simulink model "Engine_Library"  (Simulink 7.7)
settings: Solver=ode45  StartTime=0.0  StopTime=10.0  RelTol=1e-3
PostLoadFcn:
  | %%% BEGIN C7_225HP_D_HF CODE %%%
  | % Import the data from Excel for a lookup table
  | data = xlsread('Engine_Specification.xlsx', 'C7_225HP_D');
  | % Row indices for lookup table
  | breakpoints1 = data(2:end,1)';
  | % Column indices for lookup table
  | breakpoints2 = data(1,2:end);
  | % Output values for lookup table
  | table_data = data(2:end,2:end);
  | Engine_C7_225HP_D_RPM_raw = table_data(:,1);
  | Engine_C7_225HP_D_Torque_raw = table_data(:,3);
  | Engine_C7_225HP_D_Power_raw = table_data(:,2);
  | Engine_C7_225HP_D_sfc_raw = table_data(:,4);
  | Engine_C7_225HP_D_ne_raw = table_data(:,5);
  | %%% END C7_225HP_D_HF CODE %%%%%% BEGIN C9_350HP_D_HF CODE %%%
  | % Import the data from Excel for a lookup table
  | data = xlsread('Engine_Specification.xlsx', 'C9_350HP_D');
  | % Row indices for lookup table
  | breakpoints1 = data(2:end,1)';
  | % Column indices for lookup table
  | breakpoints2 = data(1,2:end);
  | % Output values for lookup table
  | table_data = data(2:end,2:end);
  | Engine_C9_350HP_D_RPM_raw = table_data(:,1);
  | Engine_C9_350HP_D_Torque_raw = table_data(:,3);
  | Engine_C9_350HP_D_Power_raw = table_data(:,2);
  | Engine_C9_350HP_D_sfc_raw = table_data(:,4);
  | Engine_C9_350HP_D_ne_raw = table_data(:,5);
  | %%% END C9_350HP_D_HF CODE %%%%%% BEGIN C13_475HP_D_HF CODE %%%
  | % Import the data from Excel for a lookup table
  | data = xlsread('Engine_Specification.xlsx', 'C13_475HP_D');
  | % Row indices for lookup table
  | breakpoints1 = data(2:end,1)';
  | % Column indices for lookup table
  | breakpoints2 = data(1,2:end);
  | % Output values for lookup table
  | table_data = data(2:end,2:end);
  | Engine_C13_475HP_D_RPM_raw = table_data(:,1);
  | Engine_C13_475HP_D_Torque_raw = table_data(:,3);
  | Engine_C13_475HP_D_Power_raw = table_data(:,2);
  | Engine_C13_475HP_D_sfc_raw = table_data(:,4);
  | Engine_C13_475HP_D_ne_raw = table_data(:,5);
  | %%% END C13_475HP_D_HF CODE %%%%%% BEGIN C15_600HP_D_HF CODE %%%
  | % Import the data from Excel for a lookup table
  | data = xlsread('Engine_Specification.xlsx', 'C15_600HP_D');
  | % Row indices for lookup table
  | breakpoints1 = data(2:end,1)';
  | % Column indices for lookup table
  | breakpoints2 = data(1,2:end);
  | % Output values for lookup table
  | table_data = data(2:end,2:end);
  | Engine_C15_600HP_D_RPM_raw = table_data(:,1);
  | Engine_C15_600HP_D_Torque_raw = table_data(:,3);
  | Engine_C15_600HP_D_Power_raw = table_data(:,2);
  | Engine_C15_600HP_D_sfc_raw = table_data(:,4);
  | Engine_C15_600HP_D_ne_raw = table_data(:,5);
  | %%% END C15_600HP_D_HF CODE %%%%%% BEGIN C7_230HP_LEFT CODE %%%
  | % Import the data from Excel for a lookup table
  | data = xlsread('Engine_Specification.xlsx', 'C7_230HP_LEFT');
  | % Row indices for lookup table
  | breakpoints1 = data(2:end,1)';
  | % Column indices for lookup table
  | breakpoints2 = data(1,2:end);
  | % Output values for lookup table
  | table_data = data(2:end,2:end);
  | Engine_C7_230HP_LEFT_RPM_raw = table_data(:,1);
  | Engine_C7_230HP_LEFT_Torque_raw = table_data(:,3);
  | Engine_C7_230HP_LEFT_Power_raw = table_data(:,2);
  | Engine_C7_230HP_LEFT_sfc_raw = table_data(:,4);
  | Engine_C7_230HP_LEFT_ne_raw = table_data(:,5);
  | %%% END C7_230HP_LEFT CODE %%%%%% BEGIN C9_COM_350HP CODE %%%
  | % Import the data from Excel for a lookup table
  | data = xlsread('Engine_Specification.xlsx', 'C9_COM_350HP');
  | % Row indices for lookup table
  | breakpoints1 = data(2:end,1)';
  | % Column indices for lookup table
  | breakpoints2 = data(1,2:end);
  | % Output values for lookup table
  | table_data = data(2:end,2:end);
  | Engine_C9_COM_350HP_RPM_raw = table_data(:,1);
  | Engine_C9_COM_350HP_Torque_raw = table_data(:,3);
  | Engine_C9_COM_350HP_Power_raw = table_data(:,2);
  | Engine_C9_COM_350HP_sfc_raw = table_data(:,4);
  | %%% END C9_COM_350HP CODE %%%%%% BEGIN C13_COM_430HP CODE %%%
  | % Import the data from Excel for a lookup table
  | data = xlsread('Engine_Specification.xlsx', 'C13_COM_430HP');
  | % Row indices for lookup table
  | breakpoints1 = data(2:end,1)';
  | % Column indices for lookup table
  | breakpoints2 = data(1,2:end);
  | % Output values for lookup table
  | table_data = data(2:end,2:end);
  | Engine_C13_COM_430HP_RPM_raw = table_data(:,1);
  | Engine_C13_COM_430HP_Torque_raw = table_data(:,3);
  | Engine_C13_COM_430HP_Power_raw = table_data(:,2);
  | Engine_C13_COM_430HP_sfc_raw = table_data(:,4);
  | %%% END C13_COM_430HP CODE %%%
libraries: simulink x3
settings Model: Creator=Zsolt  LastModifiedBy=jscott
settings HardwareCC: TargetIntDivRoundTo=Zero  TargetEndianess=LittleEndian  TargetHWDeviceType=MATLAB Host  ProdEqTarget=off
settings RTWCC: SystemTargetFile=rsim.tlc  TemplateMakefile=rsim_default_tmf  Description=Rapid Simulation Target  ProcessScript=rsim_make_rtw_hook
settings RSimTargetCC: TargetFunctionLibrary=ANSI_C  ERTMultiwordTypeDef=System defined  FunctionExecutionProfile=off  CodeExecutionProfiling=off  ERTCodeCoverageTool=None  ERTMultiwordLength=256  IsPILTarget=off  EnableShiftOperators=on  PortableWordSizes=off

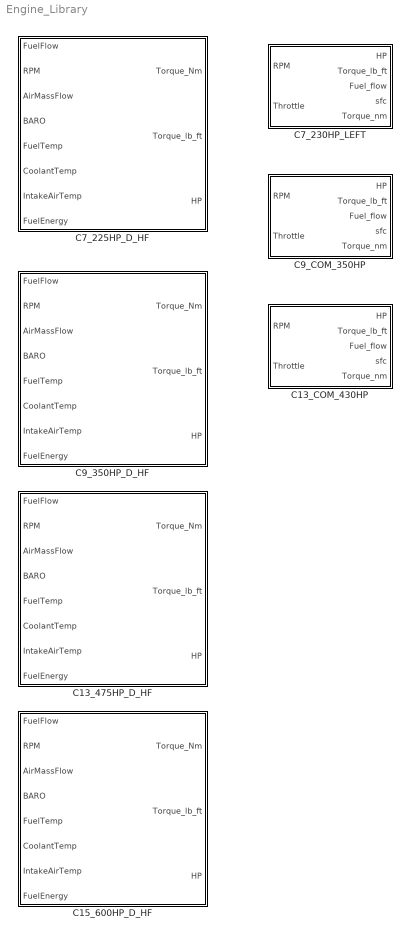
== system Engine_Library ==
  C13_475HP_D_HF : Subsystem
  C13_COM_430HP : Subsystem
  C15_600HP_D_HF : Subsystem
  C7_225HP_D_HF : Subsystem
  C7_230HP_LEFT : Subsystem
  C9_350HP_D_HF : Subsystem
  C9_COM_350HP : Subsystem

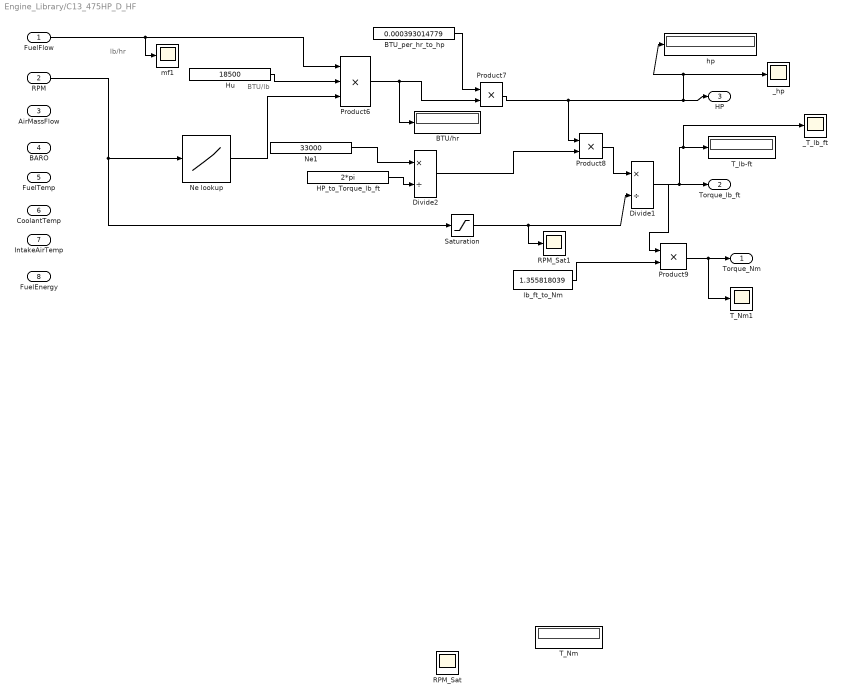
== system Engine_Library/C13_475HP_D_HF ==
  note: lb/hr
  note: BTU/lb
  FuelFlow : Inport
  RPM : Inport  Port=2
  AirMassFlow : Inport  Port=3
  BARO : Inport  Port=4
  FuelTemp : Inport  Port=5
  CoolantTemp : Inport  Port=6
  IntakeAirTemp : Inport  Port=7
  FuelEnergy : Inport  Port=8
  BTU/hr : Display
  BTU_per_hr_to_hp : Constant  Value=0.000393014779
  Divide1 : Product  Inputs=*/
  Divide2 : Product  Inputs=*/
  HP_to_Torque_lb_ft : Constant  Value=2*pi
  Hu : Constant  Value=18500
  Ne lookup : Lookup  InputValues=Engine_C13_475HP_D_RPM_raw  Table=Engine_C13_475HP_D_ne_raw
  Ne1 : Constant  Value=33000
  Product6 : Product  Inputs=3  RndMeth=Zero
  Product7 : Product  RndMeth=Zero
  Product8 : Product  RndMeth=Zero
  Product9 : Product  RndMeth=Zero
  RPM_Sat : Scope
      settings: TimeRange=100  SaveName=ScopeData4
  RPM_Sat1 : Scope
      settings: TimeRange=100  SaveName=ScopeData7
  Saturation : Saturate  UpperLimit=2100  LowerLimit=600
  T_Nm : Display
  T_Nm1 : Scope
      settings: TimeRange=100  SaveName=ScopeData6
  T_lb-ft : Display
  _T_lb_ft : Scope
      settings: SaveName=ScopeData5
  _hp : Scope
      settings: SaveName=ScopeData3
  hp : Display
  lb_ft_to_Nm : Constant  Value=1.355818039
  mf1 : Scope
      settings: SaveName=ScopeData8
  Torque_Nm : Outport
  Torque_lb_ft : Outport  Port=2
  HP : Outport  Port=3
  wires:
  FuelFlow/1 -> Product6/1, mf1/1
  Hu/1 -> Product6/2
  HP_to_Torque_lb_ft/1 -> Divide2/2
  Ne1/1 -> Divide2/1
  BTU_per_hr_to_hp/1 -> Product7/1
  Product7/1 -> Product8/1, HP/1, _hp/1, hp/1
  Product6/1 -> Product7/2, BTU/hr/1
  Divide2/1 -> Product8/2
  lb_ft_to_Nm/1 -> Product9/2
  Divide1/1 -> Torque_lb_ft/1, Product9/1, T_lb-ft/1, _T_lb_ft/1
  Product8/1 -> Divide1/1
  Saturation/1 -> Divide1/2, RPM_Sat1/1
  Product9/1 -> Torque_Nm/1, T_Nm1/1
  RPM/1 -> Saturation/1, Ne lookup/1
  Ne lookup/1 -> Product6/3

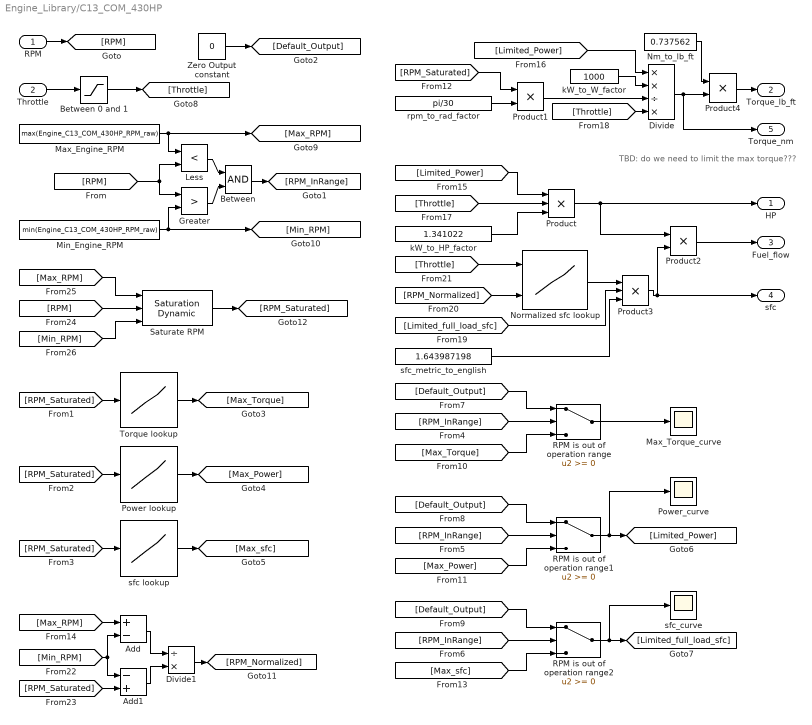
== system Engine_Library/C13_COM_430HP ==
  note: TBD: do we need to limit the max torque???
  RPM : Inport
  Throttle : Inport  Port=2
  Add : Sum  Inputs=+-
  Add1 : Sum  Inputs=-+
  Between : Logic  AllPortsSameDT=off  OutDataTypeStr=boolean
  Between 0 and 1 : Saturate  UpperLimit=1  LowerLimit=0
  Divide : Product  Inputs=**/*
  Divide1 : Product  Inputs=/*
  Greater : RelationalOperator  Operator=>  OutDataTypeStr=boolean
  Less : RelationalOperator  Operator=<  OutDataTypeStr=boolean
  Max_Engine_RPM : Constant  Value=max(Engine_C13_COM_430HP_RPM_raw)
  Max_Torque_curve : Scope
      settings: TimeRange=10  YMin=500  YMax=1000
  Min_Engine_RPM : Constant  Value=min(Engine_C13_COM_430HP_RPM_raw)
  Nm_to_lb_ft : Constant  Value=0.737562
  Normalized sfc lookup : Lookup2D  RowIndex=[0,0.25,0.5,0.75,1]  ColumnIndex=[0,0.25,0.5,0.75,1]  Table=[ 1.3562, 1.1898, 1.0652, 1.0227, 1.0000; 1.3918, 1.2098, 1.0718, 1.0316, 1.0000; 1.4074, 1.2248, 1.0865, 1.0461, 1.0000; 1.4502, 1.2557, 1.1108, 1.0540, 1.0000; 1.4127, 1.2404, 1.1120, 1.0628, 1.0000]'  LookUpMeth=Interpolation-Use End Values
  Power lookup : Lookup  InputValues=Engine_C13_COM_430HP_RPM_raw  Table=Engine_C13_COM_430HP_Power_raw
  Power_curve : Scope
      settings: TimeRange=10  YMin=50  YMax=250
  Product : Product  Inputs=3  RndMeth=Zero
  Product1 : Product  RndMeth=Zero
  Product2 : Product  RndMeth=Zero
  Product3 : Product  Inputs=3  RndMeth=Zero
  Product4 : Product  RndMeth=Zero
  RPM is out of operation range : Switch
  RPM is out of operation range1 : Switch
  RPM is out of operation range2 : Switch
  Saturate RPM : simulink/Discontinuities/Saturation Dynamic  SystemSampleTime=-1  OutMin=[]  OutMax=[]  OutDataTypeStr=Inherit: Same as second input  OutDataType=fixdt(1, 16)  OutScaling=2^-10  DoSatur=off
  Torque lookup : Lookup  InputValues=Engine_C13_COM_430HP_RPM_raw  Table=Engine_C13_COM_430HP_Torque_raw
  Zero Output constant : Constant  Value=0
  kW_to_HP_factor : Constant  Value=1.341022
  kW_to_W_factor : Constant  Value=1000
  rpm_to_rad_factor : Constant  Value=pi/30
  sfc lookup : Lookup  InputValues=Engine_C13_COM_430HP_RPM_raw  Table=Engine_C13_COM_430HP_sfc_raw
  sfc_curve : Scope
      settings: TimeRange=10  YMin=40  YMax=120  SaveName=ScopeData2
  sfc_metric_to_english : Constant  Value=1.643987198
  HP : Outport
  Torque_lb_ft : Outport  Port=2
  Fuel_flow : Outport  Port=3
  sfc : Outport  Port=4
  Torque_nm : Outport  Port=5
  wires:
  Power lookup/1 -> [Max_Power]
  sfc lookup/1 -> [Max_sfc]
  Torque lookup/1 -> [Max_Torque]
  Max_Engine_RPM/1 -> Less/1, [Max_RPM]
  RPM is out of operation range/1 -> Max_Torque_curve/1
  Throttle/1 -> Between 0 and 1/1
  kW_to_HP_factor/1 -> Product/3
  Product/1 -> HP/1, Product2/1
  rpm_to_rad_factor/1 -> Product1/2
  Product1/1 -> Divide/3
  kW_to_W_factor/1 -> Divide/2
  Product2/1 -> Fuel_flow/1
  RPM/1 -> [RPM]
  [RPM] -> Less/2, Greater/1
  [RPM_Saturated] -> Torque lookup/1
  [RPM_Saturated] -> Power lookup/1
  [RPM_Saturated] -> sfc lookup/1
  [RPM_InRange] -> RPM is out of operation range/2
  [RPM_InRange] -> RPM is out of operation range1/2
  [RPM_InRange] -> RPM is out of operation range2/2
  Zero Output constant/1 -> [Default_Output]
  [Default_Output] -> RPM is out of operation range/1
  [Default_Output] -> RPM is out of operation range1/1
  [Default_Output] -> RPM is out of operation range2/1
  [Max_Torque] -> RPM is out of operation range/3
  [Max_Power] -> RPM is out of operation range1/3
  [RPM_Saturated] -> Product1/1
  [Max_sfc] -> RPM is out of operation range2/3
  RPM is out of operation range1/1 -> [Limited_Power], Power_curve/1
  RPM is out of operation range2/1 -> [Limited_full_load_sfc], sfc_curve/1
  [Limited_Power] -> Product/1
  [Limited_Power] -> Divide/1
  Between 0 and 1/1 -> [Throttle]
  [Throttle] -> Product/2
  [Throttle] -> Divide/4
  Min_Engine_RPM/1 -> Greater/2, [Min_RPM]
  Less/1 -> Between/1
  Greater/1 -> Between/2
  Between/1 -> [RPM_InRange]
  Normalized sfc lookup/1 -> Product3/1
  [Limited_full_load_sfc] -> Product3/2
  sfc_metric_to_english/1 -> Product3/3
  Product3/1 -> sfc/1, Product2/2
  [Max_RPM] -> Add/1
  [Min_RPM] -> Add/2, Add1/1
  [RPM_Saturated] -> Add1/2
  Add/1 -> Divide1/1
  Add1/1 -> Divide1/2
  Divide1/1 -> [RPM_Normalized]
  [Throttle] -> Normalized sfc lookup/1
  [RPM_Normalized] -> Normalized sfc lookup/2
  [RPM] -> Saturate RPM/2
  [Max_RPM] -> Saturate RPM/1
  [Min_RPM] -> Saturate RPM/3
  Saturate RPM/1 -> [RPM_Saturated]
  Divide/1 -> Torque_nm/1, Product4/2
  Product4/1 -> Torque_lb_ft/1
  Nm_to_lb_ft/1 -> Product4/1

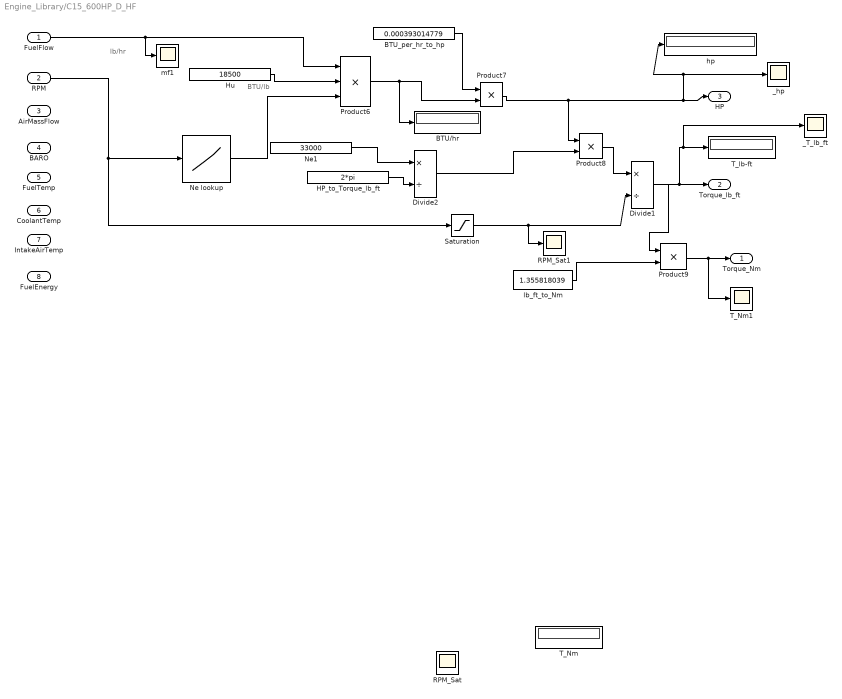
== system Engine_Library/C15_600HP_D_HF ==
  note: lb/hr
  note: BTU/lb
  FuelFlow : Inport
  RPM : Inport  Port=2
  AirMassFlow : Inport  Port=3
  BARO : Inport  Port=4
  FuelTemp : Inport  Port=5
  CoolantTemp : Inport  Port=6
  IntakeAirTemp : Inport  Port=7
  FuelEnergy : Inport  Port=8
  BTU/hr : Display
  BTU_per_hr_to_hp : Constant  Value=0.000393014779
  Divide1 : Product  Inputs=*/
  Divide2 : Product  Inputs=*/
  HP_to_Torque_lb_ft : Constant  Value=2*pi
  Hu : Constant  Value=18500
  Ne lookup : Lookup  InputValues=Engine_C15_600HP_D_RPM_raw  Table=Engine_C15_600HP_D_ne_raw
  Ne1 : Constant  Value=33000
  Product6 : Product  Inputs=3  RndMeth=Zero
  Product7 : Product  RndMeth=Zero
  Product8 : Product  RndMeth=Zero
  Product9 : Product  RndMeth=Zero
  RPM_Sat : Scope
      settings: TimeRange=100  SaveName=ScopeData4
  RPM_Sat1 : Scope
      settings: TimeRange=100  SaveName=ScopeData7
  Saturation : Saturate  UpperLimit=2100  LowerLimit=600
  T_Nm : Display
  T_Nm1 : Scope
      settings: TimeRange=100  SaveName=ScopeData6
  T_lb-ft : Display
  _T_lb_ft : Scope
      settings: SaveName=ScopeData5
  _hp : Scope
      settings: SaveName=ScopeData3
  hp : Display
  lb_ft_to_Nm : Constant  Value=1.355818039
  mf1 : Scope
      settings: SaveName=ScopeData8
  Torque_Nm : Outport
  Torque_lb_ft : Outport  Port=2
  HP : Outport  Port=3
  wires:
  FuelFlow/1 -> Product6/1, mf1/1
  Hu/1 -> Product6/2
  HP_to_Torque_lb_ft/1 -> Divide2/2
  Ne1/1 -> Divide2/1
  BTU_per_hr_to_hp/1 -> Product7/1
  Product7/1 -> Product8/1, HP/1, _hp/1, hp/1
  Product6/1 -> Product7/2, BTU/hr/1
  Divide2/1 -> Product8/2
  lb_ft_to_Nm/1 -> Product9/2
  Divide1/1 -> Torque_lb_ft/1, Product9/1, T_lb-ft/1, _T_lb_ft/1
  Product8/1 -> Divide1/1
  Saturation/1 -> Divide1/2, RPM_Sat1/1
  Product9/1 -> Torque_Nm/1, T_Nm1/1
  RPM/1 -> Saturation/1, Ne lookup/1
  Ne lookup/1 -> Product6/3

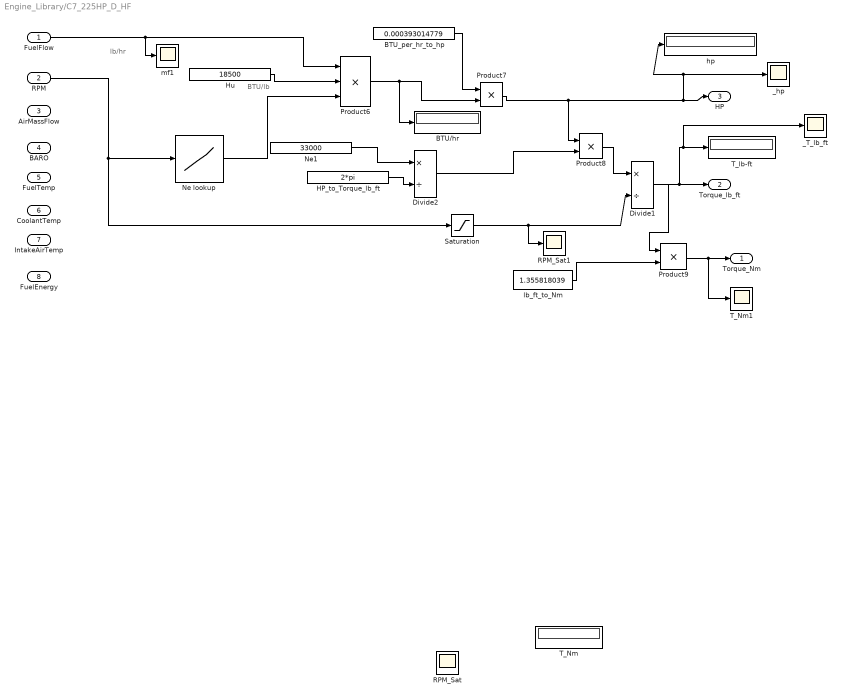
== system Engine_Library/C7_225HP_D_HF ==
  note: lb/hr
  note: BTU/lb
  FuelFlow : Inport
  RPM : Inport  Port=2
  AirMassFlow : Inport  Port=3
  BARO : Inport  Port=4
  FuelTemp : Inport  Port=5
  CoolantTemp : Inport  Port=6
  IntakeAirTemp : Inport  Port=7
  FuelEnergy : Inport  Port=8
  BTU/hr : Display
  BTU_per_hr_to_hp : Constant  Value=0.000393014779
  Divide1 : Product  Inputs=*/
  Divide2 : Product  Inputs=*/
  HP_to_Torque_lb_ft : Constant  Value=2*pi
  Hu : Constant  Value=18500
  Ne lookup : Lookup  InputValues=Engine_C7_225HP_D_RPM_raw  Table=Engine_C7_225HP_D_ne_raw
  Ne1 : Constant  Value=33000
  Product6 : Product  Inputs=3  RndMeth=Zero
  Product7 : Product  RndMeth=Zero
  Product8 : Product  RndMeth=Zero
  Product9 : Product  RndMeth=Zero
  RPM_Sat : Scope
      settings: TimeRange=100  SaveName=ScopeData4
  RPM_Sat1 : Scope
      settings: TimeRange=100  SaveName=ScopeData7
  Saturation : Saturate  UpperLimit=2500  LowerLimit=600
  T_Nm : Display
  T_Nm1 : Scope
      settings: TimeRange=100  SaveName=ScopeData6
  T_lb-ft : Display
  _T_lb_ft : Scope
      settings: SaveName=ScopeData5
  _hp : Scope
      settings: SaveName=ScopeData3
  hp : Display
  lb_ft_to_Nm : Constant  Value=1.355818039
  mf1 : Scope
      settings: SaveName=ScopeData8
  Torque_Nm : Outport
  Torque_lb_ft : Outport  Port=2
  HP : Outport  Port=3
  wires:
  FuelFlow/1 -> Product6/1, mf1/1
  Hu/1 -> Product6/2
  HP_to_Torque_lb_ft/1 -> Divide2/2
  Ne1/1 -> Divide2/1
  BTU_per_hr_to_hp/1 -> Product7/1
  Product7/1 -> Product8/1, HP/1, _hp/1, hp/1
  Product6/1 -> Product7/2, BTU/hr/1
  Divide2/1 -> Product8/2
  lb_ft_to_Nm/1 -> Product9/2
  Divide1/1 -> Torque_lb_ft/1, Product9/1, T_lb-ft/1, _T_lb_ft/1
  Product8/1 -> Divide1/1
  Saturation/1 -> Divide1/2, RPM_Sat1/1
  Product9/1 -> Torque_Nm/1, T_Nm1/1
  RPM/1 -> Saturation/1, Ne lookup/1
  Ne lookup/1 -> Product6/3

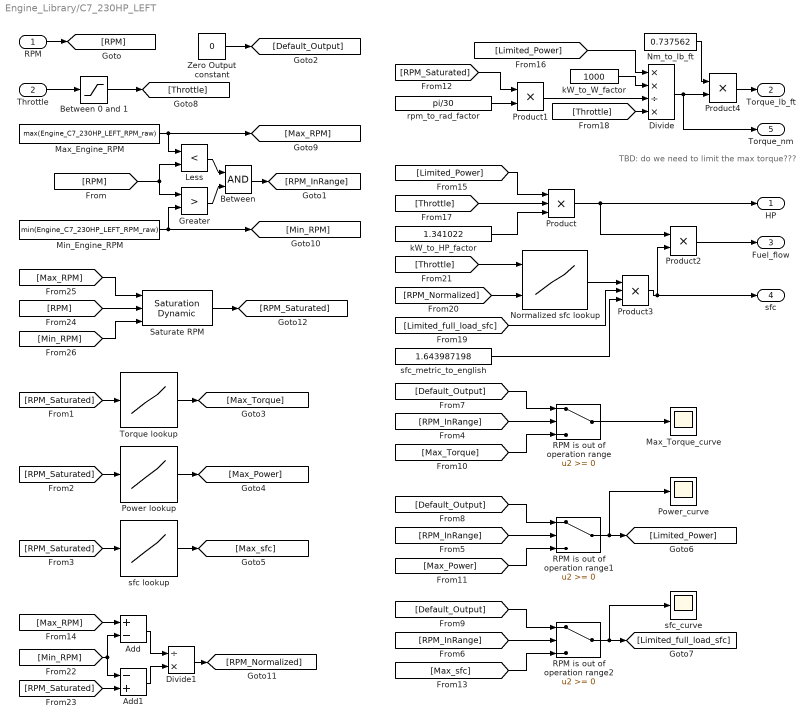
== system Engine_Library/C7_230HP_LEFT ==
  note: TBD: do we need to limit the max torque???
  RPM : Inport
  Throttle : Inport  Port=2
  Add : Sum  Inputs=+-
  Add1 : Sum  Inputs=-+
  Between : Logic  AllPortsSameDT=off  OutDataTypeStr=boolean
  Between 0 and 1 : Saturate  UpperLimit=1  LowerLimit=0
  Divide : Product  Inputs=**/*
  Divide1 : Product  Inputs=/*
  Greater : RelationalOperator  Operator=>  OutDataTypeStr=boolean
  Less : RelationalOperator  Operator=<  OutDataTypeStr=boolean
  Max_Engine_RPM : Constant  Value=max(Engine_C7_230HP_LEFT_RPM_raw)
  Max_Torque_curve : Scope
      settings: TimeRange=10  YMin=500  YMax=1000
  Min_Engine_RPM : Constant  Value=min(Engine_C7_230HP_LEFT_RPM_raw)
  Nm_to_lb_ft : Constant  Value=0.737562
  Normalized sfc lookup : Lookup2D  RowIndex=[0,0.25,0.5,0.75,1]  ColumnIndex=[0,0.25,0.5,0.75,1]  Table=[ 1.3562, 1.1898, 1.0652, 1.0227, 1.0000; 1.3918, 1.2098, 1.0718, 1.0316, 1.0000; 1.4074, 1.2248, 1.0865, 1.0461, 1.0000; 1.4502, 1.2557, 1.1108, 1.0540, 1.0000; 1.4127, 1.2404, 1.1120, 1.0628, 1.0000]'  LookUpMeth=Interpolation-Use End Values
  Power lookup : Lookup  InputValues=Engine_C7_230HP_LEFT_RPM_raw  Table=Engine_C7_230HP_LEFT_Power_raw
  Power_curve : Scope
      settings: TimeRange=10  YMin=50  YMax=250
  Product : Product  Inputs=3  RndMeth=Zero
  Product1 : Product  RndMeth=Zero
  Product2 : Product  RndMeth=Zero
  Product3 : Product  Inputs=3  RndMeth=Zero
  Product4 : Product  RndMeth=Zero
  RPM is out of operation range : Switch
  RPM is out of operation range1 : Switch
  RPM is out of operation range2 : Switch
  Saturate RPM : simulink/Discontinuities/Saturation Dynamic  SystemSampleTime=-1  OutMin=[]  OutMax=[]  OutDataTypeStr=Inherit: Same as second input  OutDataType=fixdt(1, 16)  OutScaling=2^-10  DoSatur=off
  Torque lookup : Lookup  InputValues=Engine_C7_230HP_LEFT_RPM_raw  Table=Engine_C7_230HP_LEFT_Torque_raw
  Zero Output constant : Constant  Value=0
  kW_to_HP_factor : Constant  Value=1.341022
  kW_to_W_factor : Constant  Value=1000
  rpm_to_rad_factor : Constant  Value=pi/30
  sfc lookup : Lookup  InputValues=Engine_C7_230HP_LEFT_RPM_raw  Table=Engine_C7_230HP_LEFT_sfc_raw
  sfc_curve : Scope
      settings: TimeRange=10  YMin=40  YMax=120  SaveName=ScopeData2
  sfc_metric_to_english : Constant  Value=1.643987198
  HP : Outport
  Torque_lb_ft : Outport  Port=2
  Fuel_flow : Outport  Port=3
  sfc : Outport  Port=4
  Torque_nm : Outport  Port=5
  wires:
  Power lookup/1 -> [Max_Power]
  sfc lookup/1 -> [Max_sfc]
  Torque lookup/1 -> [Max_Torque]
  Max_Engine_RPM/1 -> Less/1, [Max_RPM]
  RPM is out of operation range/1 -> Max_Torque_curve/1
  Throttle/1 -> Between 0 and 1/1
  kW_to_HP_factor/1 -> Product/3
  Product/1 -> HP/1, Product2/1
  rpm_to_rad_factor/1 -> Product1/2
  Product1/1 -> Divide/3
  kW_to_W_factor/1 -> Divide/2
  Product2/1 -> Fuel_flow/1
  RPM/1 -> [RPM]
  [RPM] -> Less/2, Greater/1
  [RPM_Saturated] -> Torque lookup/1
  [RPM_Saturated] -> Power lookup/1
  [RPM_Saturated] -> sfc lookup/1
  [RPM_InRange] -> RPM is out of operation range/2
  [RPM_InRange] -> RPM is out of operation range1/2
  [RPM_InRange] -> RPM is out of operation range2/2
  Zero Output constant/1 -> [Default_Output]
  [Default_Output] -> RPM is out of operation range/1
  [Default_Output] -> RPM is out of operation range1/1
  [Default_Output] -> RPM is out of operation range2/1
  [Max_Torque] -> RPM is out of operation range/3
  [Max_Power] -> RPM is out of operation range1/3
  [RPM_Saturated] -> Product1/1
  [Max_sfc] -> RPM is out of operation range2/3
  RPM is out of operation range1/1 -> [Limited_Power], Power_curve/1
  RPM is out of operation range2/1 -> [Limited_full_load_sfc], sfc_curve/1
  [Limited_Power] -> Product/1
  [Limited_Power] -> Divide/1
  Between 0 and 1/1 -> [Throttle]
  [Throttle] -> Product/2
  [Throttle] -> Divide/4
  Min_Engine_RPM/1 -> Greater/2, [Min_RPM]
  Less/1 -> Between/1
  Greater/1 -> Between/2
  Between/1 -> [RPM_InRange]
  Normalized sfc lookup/1 -> Product3/1
  [Limited_full_load_sfc] -> Product3/2
  sfc_metric_to_english/1 -> Product3/3
  Product3/1 -> sfc/1, Product2/2
  [Max_RPM] -> Add/1
  [Min_RPM] -> Add/2, Add1/1
  [RPM_Saturated] -> Add1/2
  Add/1 -> Divide1/1
  Add1/1 -> Divide1/2
  Divide1/1 -> [RPM_Normalized]
  [Throttle] -> Normalized sfc lookup/1
  [RPM_Normalized] -> Normalized sfc lookup/2
  [RPM] -> Saturate RPM/2
  [Max_RPM] -> Saturate RPM/1
  [Min_RPM] -> Saturate RPM/3
  Saturate RPM/1 -> [RPM_Saturated]
  Divide/1 -> Torque_nm/1, Product4/2
  Product4/1 -> Torque_lb_ft/1
  Nm_to_lb_ft/1 -> Product4/1

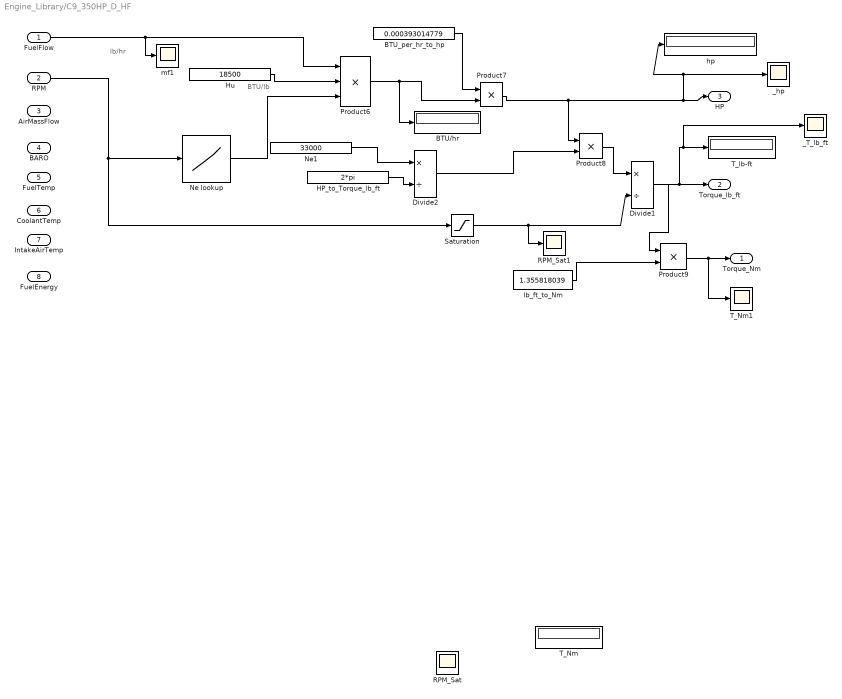
== system Engine_Library/C9_350HP_D_HF ==
  note: lb/hr
  note: BTU/lb
  FuelFlow : Inport
  RPM : Inport  Port=2
  AirMassFlow : Inport  Port=3
  BARO : Inport  Port=4
  FuelTemp : Inport  Port=5
  CoolantTemp : Inport  Port=6
  IntakeAirTemp : Inport  Port=7
  FuelEnergy : Inport  Port=8
  BTU/hr : Display
  BTU_per_hr_to_hp : Constant  Value=0.000393014779
  Divide1 : Product  Inputs=*/
  Divide2 : Product  Inputs=*/
  HP_to_Torque_lb_ft : Constant  Value=2*pi
  Hu : Constant  Value=18500
  Ne lookup : Lookup  InputValues=Engine_C9_350HP_D_RPM_raw  Table=Engine_C9_350HP_D_ne_raw
  Ne1 : Constant  Value=33000
  Product6 : Product  Inputs=3  RndMeth=Zero
  Product7 : Product  RndMeth=Zero
  Product8 : Product  RndMeth=Zero
  Product9 : Product  RndMeth=Zero
  RPM_Sat : Scope
      settings: TimeRange=100  SaveName=ScopeData4
  RPM_Sat1 : Scope
      settings: TimeRange=100  SaveName=ScopeData7
  Saturation : Saturate  UpperLimit=2100  LowerLimit=600
  T_Nm : Display
  T_Nm1 : Scope
      settings: TimeRange=100  SaveName=ScopeData6
  T_lb-ft : Display
  _T_lb_ft : Scope
      settings: SaveName=ScopeData5
  _hp : Scope
      settings: SaveName=ScopeData3
  hp : Display
  lb_ft_to_Nm : Constant  Value=1.355818039
  mf1 : Scope
      settings: SaveName=ScopeData8
  Torque_Nm : Outport
  Torque_lb_ft : Outport  Port=2
  HP : Outport  Port=3
  wires:
  FuelFlow/1 -> Product6/1, mf1/1
  Hu/1 -> Product6/2
  HP_to_Torque_lb_ft/1 -> Divide2/2
  Ne1/1 -> Divide2/1
  BTU_per_hr_to_hp/1 -> Product7/1
  Product7/1 -> Product8/1, HP/1, _hp/1, hp/1
  Product6/1 -> Product7/2, BTU/hr/1
  Divide2/1 -> Product8/2
  lb_ft_to_Nm/1 -> Product9/2
  Divide1/1 -> Torque_lb_ft/1, Product9/1, T_lb-ft/1, _T_lb_ft/1
  Product8/1 -> Divide1/1
  Saturation/1 -> Divide1/2, RPM_Sat1/1
  Product9/1 -> Torque_Nm/1, T_Nm1/1
  RPM/1 -> Saturation/1, Ne lookup/1
  Ne lookup/1 -> Product6/3

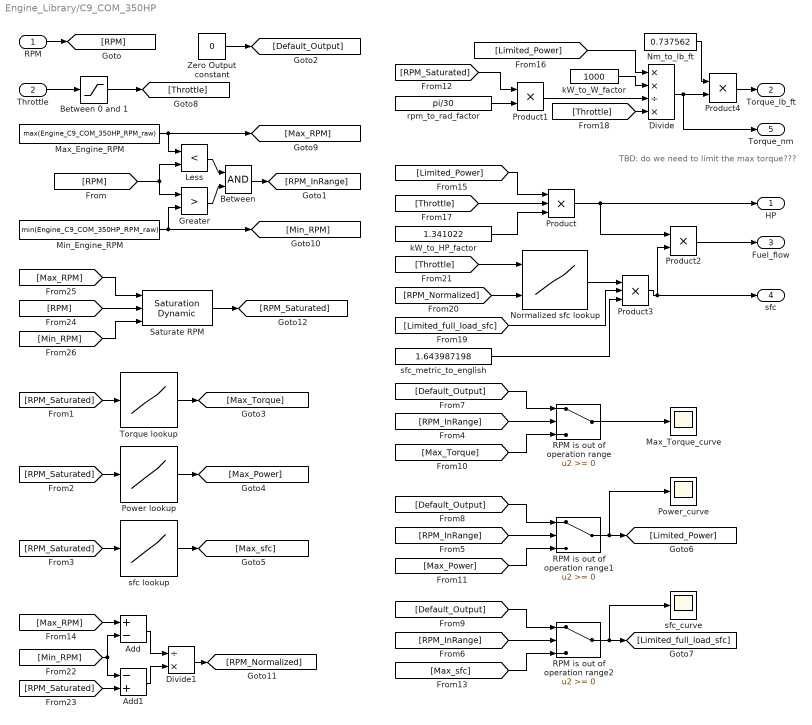
== system Engine_Library/C9_COM_350HP ==
  note: TBD: do we need to limit the max torque???
  RPM : Inport
  Throttle : Inport  Port=2
  Add : Sum  Inputs=+-
  Add1 : Sum  Inputs=-+
  Between : Logic  AllPortsSameDT=off  OutDataTypeStr=boolean
  Between 0 and 1 : Saturate  UpperLimit=1  LowerLimit=0
  Divide : Product  Inputs=**/*
  Divide1 : Product  Inputs=/*
  Greater : RelationalOperator  Operator=>  OutDataTypeStr=boolean
  Less : RelationalOperator  Operator=<  OutDataTypeStr=boolean
  Max_Engine_RPM : Constant  Value=max(Engine_C9_COM_350HP_RPM_raw)
  Max_Torque_curve : Scope
      settings: TimeRange=10  YMin=500  YMax=1000
  Min_Engine_RPM : Constant  Value=min(Engine_C9_COM_350HP_RPM_raw)
  Nm_to_lb_ft : Constant  Value=0.737562
  Normalized sfc lookup : Lookup2D  RowIndex=[0,0.25,0.5,0.75,1]  ColumnIndex=[0,0.25,0.5,0.75,1]  Table=[ 1.3562, 1.1898, 1.0652, 1.0227, 1.0000; 1.3918, 1.2098, 1.0718, 1.0316, 1.0000; 1.4074, 1.2248, 1.0865, 1.0461, 1.0000; 1.4502, 1.2557, 1.1108, 1.0540, 1.0000; 1.4127, 1.2404, 1.1120, 1.0628, 1.0000]'  LookUpMeth=Interpolation-Use End Values
  Power lookup : Lookup  InputValues=Engine_C9_COM_350HP_RPM_raw  Table=Engine_C9_COM_350HP_Power_raw
  Power_curve : Scope
      settings: TimeRange=10  YMin=50  YMax=250
  Product : Product  Inputs=3  RndMeth=Zero
  Product1 : Product  RndMeth=Zero
  Product2 : Product  RndMeth=Zero
  Product3 : Product  Inputs=3  RndMeth=Zero
  Product4 : Product  RndMeth=Zero
  RPM is out of operation range : Switch
  RPM is out of operation range1 : Switch
  RPM is out of operation range2 : Switch
  Saturate RPM : simulink/Discontinuities/Saturation Dynamic  SystemSampleTime=-1  OutMin=[]  OutMax=[]  OutDataTypeStr=Inherit: Same as second input  OutDataType=fixdt(1, 16)  OutScaling=2^-10  DoSatur=off
  Torque lookup : Lookup  InputValues=Engine_C9_COM_350HP_RPM_raw  Table=Engine_C9_COM_350HP_Torque_raw
  Zero Output constant : Constant  Value=0
  kW_to_HP_factor : Constant  Value=1.341022
  kW_to_W_factor : Constant  Value=1000
  rpm_to_rad_factor : Constant  Value=pi/30
  sfc lookup : Lookup  InputValues=Engine_C9_COM_350HP_RPM_raw  Table=Engine_C9_COM_350HP_sfc_raw
  sfc_curve : Scope
      settings: TimeRange=10  YMin=40  YMax=120  SaveName=ScopeData2
  sfc_metric_to_english : Constant  Value=1.643987198
  HP : Outport
  Torque_lb_ft : Outport  Port=2
  Fuel_flow : Outport  Port=3
  sfc : Outport  Port=4
  Torque_nm : Outport  Port=5
  wires:
  Power lookup/1 -> [Max_Power]
  sfc lookup/1 -> [Max_sfc]
  Torque lookup/1 -> [Max_Torque]
  Max_Engine_RPM/1 -> Less/1, [Max_RPM]
  RPM is out of operation range/1 -> Max_Torque_curve/1
  Throttle/1 -> Between 0 and 1/1
  kW_to_HP_factor/1 -> Product/3
  Product/1 -> HP/1, Product2/1
  rpm_to_rad_factor/1 -> Product1/2
  Product1/1 -> Divide/3
  kW_to_W_factor/1 -> Divide/2
  Product2/1 -> Fuel_flow/1
  RPM/1 -> [RPM]
  [RPM] -> Less/2, Greater/1
  [RPM_Saturated] -> Torque lookup/1
  [RPM_Saturated] -> Power lookup/1
  [RPM_Saturated] -> sfc lookup/1
  [RPM_InRange] -> RPM is out of operation range/2
  [RPM_InRange] -> RPM is out of operation range1/2
  [RPM_InRange] -> RPM is out of operation range2/2
  Zero Output constant/1 -> [Default_Output]
  [Default_Output] -> RPM is out of operation range/1
  [Default_Output] -> RPM is out of operation range1/1
  [Default_Output] -> RPM is out of operation range2/1
  [Max_Torque] -> RPM is out of operation range/3
  [Max_Power] -> RPM is out of operation range1/3
  [RPM_Saturated] -> Product1/1
  [Max_sfc] -> RPM is out of operation range2/3
  RPM is out of operation range1/1 -> [Limited_Power], Power_curve/1
  RPM is out of operation range2/1 -> [Limited_full_load_sfc], sfc_curve/1
  [Limited_Power] -> Product/1
  [Limited_Power] -> Divide/1
  Between 0 and 1/1 -> [Throttle]
  [Throttle] -> Product/2
  [Throttle] -> Divide/4
  Min_Engine_RPM/1 -> Greater/2, [Min_RPM]
  Less/1 -> Between/1
  Greater/1 -> Between/2
  Between/1 -> [RPM_InRange]
  Normalized sfc lookup/1 -> Product3/1
  [Limited_full_load_sfc] -> Product3/2
  sfc_metric_to_english/1 -> Product3/3
  Product3/1 -> sfc/1, Product2/2
  [Max_RPM] -> Add/1
  [Min_RPM] -> Add/2, Add1/1
  [RPM_Saturated] -> Add1/2
  Add/1 -> Divide1/1
  Add1/1 -> Divide1/2
  Divide1/1 -> [RPM_Normalized]
  [Throttle] -> Normalized sfc lookup/1
  [RPM_Normalized] -> Normalized sfc lookup/2
  [RPM] -> Saturate RPM/2
  [Max_RPM] -> Saturate RPM/1
  [Min_RPM] -> Saturate RPM/3
  Saturate RPM/1 -> [RPM_Saturated]
  Divide/1 -> Torque_nm/1, Product4/2
  Product4/1 -> Torque_lb_ft/1
  Nm_to_lb_ft/1 -> Product4/1
